simulink model "stm32f4_target_mpl3115a2"  (Simulink 7.3)
settings: Solver=FixedStepDiscrete  SolverMode=SingleTasking  StartTime=0.0  StopTime=1  RelTol=1e-3
PreLoadFcn:
  | waijung.modelPreload; % Required for working with Waijung Blockset. Do not remove.
undefined symbols (not defined in the file): HSEOSC, Link, LQFP176, ST, STM32F417IG
libraries: simulink x15, stm32f4_device_config_lib x1
(part 2 of 2)

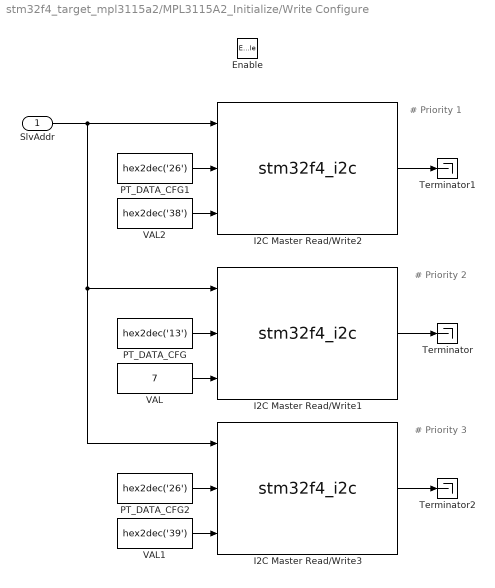
== system stm32f4_target_mpl3115a2/MPL3115A2_Initialize/Write Configure ==
  note: # Priority 1
  note: # Priority 2
  note: # Priority 3
  SlvAddr : Inport  OutDataType=fixdt(1, 16)  OutScaling=2^0
  Enable : EnablePort
  I2C Master Read/Write1 : S-Function  Priority=2  FunctionName=stm32f4_i2c  Parameters=configuration,module,transfer,clkspeed,timeout,sdapin,sclpin,writecount,readcount,inputtypearray,outputtypearray,confstr,sampletime,sampletimestr,blockid  EnableBusSupport=off  mask(stm32f4_i2c){configuration=Transaction, module=1, lastmodule=3, transfer=Blocking, dutycycle=TLow/THigh = 2, clkspeed=400, timeout=25, writecount=2, readcount=0, sdapin=C9, sclpin=A8, waitwritetime=0, inputtypearray=[3 3 3 3], outputtypearray=[1 3], confstr=["C","9","A","8","1","1","6","0","I2C_DutyCycle_2","0","off"], sampletime=-1, sampletimestr=1, blockid=MPL3115A2_InitializeWriteConfigureI2CMasterReadWrite1}
      mask prompts: module "I2C Module"; lastmodule "Last module"; transfer "Transfer mode"; dutycycle "Duty cycle in fast mode"; clkspeed "Clock speed (kHz)"; timeout "Timeout (ms)"; writecount "Bytes write count"; readcount "Bytes read count"; sdapin "SDA pin"; sclpin "SCL pin"; waitwritetime "Wait write time (ms), default is 0"; inputtypearray "Input type array"; outputtypearray "Output type array"; confstr "Configuration string"; sampletime "Sample time (sec)"; sampletimestr "Compiled sample time (sec) in string"
      mask init:
      | stm32f4_i2c_callback('init');
      mask Help: web(fullfile(waijungdocroot,'stm32f4_i2c_readwrite.htm'), '-browser')
      mask StyleString: popup(Setup|Transaction),popup(1|2|3),edit,popup(Blocking|Non-blocking),popup(TLow/THigh = 16/9|TLow/THigh = 2),edit,edit,edit,edit,popup(-|C9),popup(-|A8),edit,edit,edit,edit,edit,edit,edit
      mask CallbackString: stm32f4_i2c_callback('configuration');|stm32f4_i2c_callback('module');|||stm32f4_i2c_callback('dutycycle');|||stm32f4_i2c_callback('writecount');|stm32f4_i2c_callback('readcount');|stm32f4_i2c_callback('sdapin');|stm32f4_i2c_callback('sclpin');||||stm32f4_i2c_callback('confstr');|stm32f4_i2c_callback('sampletime');|stm32f4_i2c_callback('sampletimestr');|stm32f4_i2c_callback('blockid');
      mask Display: text(0.5, 0.5, 'Module: I2C1\nTransfer: Blocking\nWrite: 2 bytes\nRead: 0 bytes\nTs (sec): 1','ver','middle','hor','center');port_label('input', 1,'SlvAddr');port_label('input', 2,'Wr0 (uint8)');port_label('input', 3,'Wr1 (uint8)');port_label('output', 1,'Status');
  I2C Master Read/Write2 : S-Function  Priority=1  FunctionName=stm32f4_i2c  Parameters=configuration,module,transfer,clkspeed,timeout,sdapin,sclpin,writecount,readcount,inputtypearray,outputtypearray,confstr,sampletime,sampletimestr,blockid  EnableBusSupport=off  mask(stm32f4_i2c){configuration=Transaction, module=1, lastmodule=3, transfer=Blocking, dutycycle=TLow/THigh = 2, clkspeed=400, timeout=25, writecount=2, readcount=0, sdapin=C9, sclpin=A8, waitwritetime=0, inputtypearray=[3 3 3 3], outputtypearray=[1 3], confstr=["C","9","A","8","1","1","6","0","I2C_DutyCycle_2","0","off"], sampletime=-1, sampletimestr=1, blockid=MPL3115A2_InitializeWriteConfigureI2CMasterReadWrite2}
      mask prompts: module "I2C Module"; lastmodule "Last module"; transfer "Transfer mode"; dutycycle "Duty cycle in fast mode"; clkspeed "Clock speed (kHz)"; timeout "Timeout (ms)"; writecount "Bytes write count"; readcount "Bytes read count"; sdapin "SDA pin"; sclpin "SCL pin"; waitwritetime "Wait write time (ms), default is 0"; inputtypearray "Input type array"; outputtypearray "Output type array"; confstr "Configuration string"; sampletime "Sample time (sec)"; sampletimestr "Compiled sample time (sec) in string"
      mask init:
      | stm32f4_i2c_callback('init');
      mask Help: web(fullfile(waijungdocroot,'stm32f4_i2c_readwrite.htm'), '-browser')
      mask StyleString: popup(Setup|Transaction),popup(1|2|3),edit,popup(Blocking|Non-blocking),popup(TLow/THigh = 16/9|TLow/THigh = 2),edit,edit,edit,edit,popup(-|C9),popup(-|A8),edit,edit,edit,edit,edit,edit,edit
      mask CallbackString: stm32f4_i2c_callback('configuration');|stm32f4_i2c_callback('module');|||stm32f4_i2c_callback('dutycycle');|||stm32f4_i2c_callback('writecount');|stm32f4_i2c_callback('readcount');|stm32f4_i2c_callback('sdapin');|stm32f4_i2c_callback('sclpin');||||stm32f4_i2c_callback('confstr');|stm32f4_i2c_callback('sampletime');|stm32f4_i2c_callback('sampletimestr');|stm32f4_i2c_callback('blockid');
      mask Display: text(0.5, 0.5, 'Module: I2C1\nTransfer: Blocking\nWrite: 2 bytes\nRead: 0 bytes\nTs (sec): 1','ver','middle','hor','center');port_label('input', 1,'SlvAddr');port_label('input', 2,'Wr0 (uint8)');port_label('input', 3,'Wr1 (uint8)');port_label('output', 1,'Status');
  I2C Master Read/Write3 : S-Function  Priority=3  FunctionName=stm32f4_i2c  Parameters=configuration,module,transfer,clkspeed,timeout,sdapin,sclpin,writecount,readcount,inputtypearray,outputtypearray,confstr,sampletime,sampletimestr,blockid  EnableBusSupport=off  mask(stm32f4_i2c){configuration=Transaction, module=1, lastmodule=3, transfer=Blocking, dutycycle=TLow/THigh = 2, clkspeed=400, timeout=25, writecount=2, readcount=0, sdapin=C9, sclpin=A8, waitwritetime=0, inputtypearray=[3 3 3 3], outputtypearray=[1 3], confstr=["C","9","A","8","1","1","6","0","I2C_DutyCycle_2","0","off"], sampletime=-1, sampletimestr=1, blockid=MPL3115A2_InitializeWriteConfigureI2CMasterReadWrite3}
      mask prompts: module "I2C Module"; lastmodule "Last module"; transfer "Transfer mode"; dutycycle "Duty cycle in fast mode"; clkspeed "Clock speed (kHz)"; timeout "Timeout (ms)"; writecount "Bytes write count"; readcount "Bytes read count"; sdapin "SDA pin"; sclpin "SCL pin"; waitwritetime "Wait write time (ms), default is 0"; inputtypearray "Input type array"; outputtypearray "Output type array"; confstr "Configuration string"; sampletime "Sample time (sec)"; sampletimestr "Compiled sample time (sec) in string"
      mask init:
      | stm32f4_i2c_callback('init');
      mask Help: web(fullfile(waijungdocroot,'stm32f4_i2c_readwrite.htm'), '-browser')
      mask StyleString: popup(Setup|Transaction),popup(1|2|3),edit,popup(Blocking|Non-blocking),popup(TLow/THigh = 16/9|TLow/THigh = 2),edit,edit,edit,edit,popup(-|C9),popup(-|A8),edit,edit,edit,edit,edit,edit,edit
      mask CallbackString: stm32f4_i2c_callback('configuration');|stm32f4_i2c_callback('module');|||stm32f4_i2c_callback('dutycycle');|||stm32f4_i2c_callback('writecount');|stm32f4_i2c_callback('readcount');|stm32f4_i2c_callback('sdapin');|stm32f4_i2c_callback('sclpin');||||stm32f4_i2c_callback('confstr');|stm32f4_i2c_callback('sampletime');|stm32f4_i2c_callback('sampletimestr');|stm32f4_i2c_callback('blockid');
      mask Display: text(0.5, 0.5, 'Module: I2C1\nTransfer: Blocking\nWrite: 2 bytes\nRead: 0 bytes\nTs (sec): 1','ver','middle','hor','center');port_label('input', 1,'SlvAddr');port_label('input', 2,'Wr0 (uint8)');port_label('input', 3,'Wr1 (uint8)');port_label('output', 1,'Status');
  PT_DATA_CFG : Constant  Value=hex2dec('13')  OutDataTypeMode=uint8  OutDataType=fixdt(1, 16)  OutScaling=2^0  OutDataTypeStr=uint8
  PT_DATA_CFG1 : Constant  Value=hex2dec('26')  OutDataTypeMode=uint8  OutDataType=fixdt(1, 16)  OutScaling=2^0  OutDataTypeStr=uint8
  PT_DATA_CFG2 : Constant  Value=hex2dec('26')  OutDataTypeMode=uint8  OutDataType=fixdt(1, 16)  OutScaling=2^0  OutDataTypeStr=uint8
  Terminator : Terminator
  Terminator1 : Terminator
  Terminator2 : Terminator
  VAL : Constant  Value=7  OutDataTypeMode=uint8  OutDataType=fixdt(1, 16)  OutScaling=2^0  OutDataTypeStr=uint8
  VAL1 : Constant  Value=hex2dec('39')  OutDataTypeMode=uint8  OutDataType=fixdt(1, 16)  OutScaling=2^0  OutDataTypeStr=uint8
  VAL2 : Constant  Value=hex2dec('38')  OutDataTypeMode=uint8  OutDataType=fixdt(1, 16)  OutScaling=2^0  OutDataTypeStr=uint8
  wires:
  PT_DATA_CFG/1 -> I2C Master Read/Write1/2
  SlvAddr/1 -> I2C Master Read/Write2/1, I2C Master Read/Write1/1, I2C Master Read/Write3/1
  VAL/1 -> I2C Master Read/Write1/3
  I2C Master Read/Write1/1 -> Terminator/1
  PT_DATA_CFG1/1 -> I2C Master Read/Write2/2
  VAL2/1 -> I2C Master Read/Write2/3
  I2C Master Read/Write2/1 -> Terminator1/1
  PT_DATA_CFG2/1 -> I2C Master Read/Write3/2
  VAL1/1 -> I2C Master Read/Write3/3
  I2C Master Read/Write3/1 -> Terminator2/1
